simulink model "Aufgabe_3f"  (Simulink 8.7)
settings: Solver=VariableStepAuto  StartTime=0.0  StopTime=30  RelTol=1e-3
values from neighbouring files (symbols this model uses):
  A = [0,1;0,-a]    [main.m]    (also in trajectorystates.m)
  B = [0;b]    [main.m]
  C = [1,0]    [main.m]
undefined symbols (not defined in the file or in its folder): K2, Ki2, Kp2
settings Model: Creator=Andreas  LastModifiedBy=Andreas
settings DataIOCC: LimitDataPoints=off  SaveFormat=Dataset
settings DebuggingCC: UnderspecifiedInitializationDetection=Simplified  MergeDetectMultiDrivingBlocksExec=error
settings HardwareCC: ProdBitPerPointer=64  ProdLargestAtomicFloat=Float  ProdIntDivRoundTo=Zero  ProdEndianess=LittleEndian  ProdWordSize=64  ProdHWDeviceType=Intel->x86-64 (Windows64)
settings ModelReferenceCC: PropagateSignalLabelsOutOfModel=on
settings ConfigComp: CovModelRefEnable=off

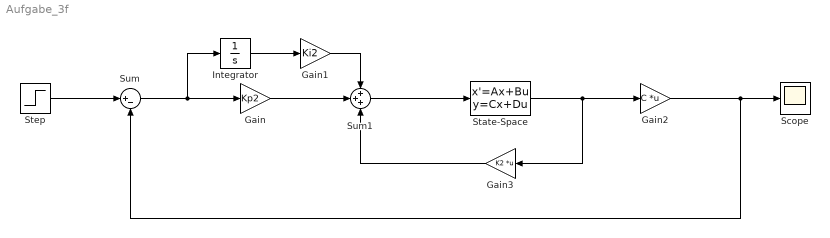
== system Aufgabe_3f ==
  Gain : Gain  Gain=Kp2
  Gain1 : Gain  Gain=Ki2
  Gain2 : Gain  Gain=C  Multiplication=Matrix(K*u)
  Gain3 : Gain  Gain=K2  Multiplication=Matrix(K*u)
  Integrator : Integrator
  Scope : Scope
  State-Space : StateSpace  A=A  B=B  C=eye(2)  D=[0;0]  X0=0
  Step : Step  Time=0  After=4*pi  SampleTime=0
  Sum : Sum  Inputs=|+-
  Sum1 : Sum  Inputs=+++
  wires:
  Step/1 -> Sum/1
  Sum/1 -> Integrator/1, Gain/1
  Gain/1 -> Sum1/2
  Integrator/1 -> Gain1/1
  Gain1/1 -> Sum1/1
  Sum1/1 -> State-Space/1
  State-Space/1 -> Gain3/1, Gain2/1
  Gain2/1 -> Sum/2, Scope/1
  Gain3/1 -> Sum1/3
